simulink model "PV_validation"  (R2020a)
settings: Solver=VariableStepAuto  StartTime=0.0  StopTime=10  RelTol=1e-3
values from neighbouring files (symbols this model uses):
  Ts = 10e-6    (= 1e-05)    [run_validation.m]    (also in tune_inverter_GFL.m; tune_inverter_PV_GFL.m; tune_iter_GFL.m = tsim(2)-tsim(1); tune_iter_PV_GFL.m = tsim(2)-tsim(1))
libraries: powerlib x6, libFC_PV x1
settings Model: SimulationMode=accelerator  Creator=pkoralew  LastModifiedBy=pkoralew

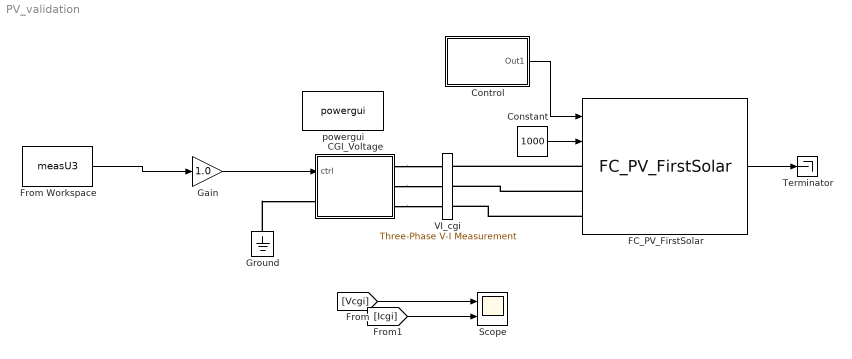
== system PV_validation ==
  CGI_Voltage : Subsystem
  Constant : Constant  Value=1000
  Control : Subsystem
  FC_PV_FirstSolar : libFC_PV/FC_PV_FirstSolar  EnArray=off  Ts=Ts  cc_kp=-1  cc_Ti=-1  pll_kp=-1  pll_ki=-1
  From Workspace : FromWorkspace  VariableName=measU3  SampleTime=Ts
  Gain : Gain  Gain=1.0
  Ground : powerlib/Elements/Ground  LConnTagsString=a
  Scope : Scope  NumInputPorts=2
  Terminator : Terminator
  VI_cgi : powerlib/Measurements/Three-Phase V-I Measurement  VoltageMeasurement=phase-to-ground  SetLabelV=on  LabelV=Vcgi  Vpu=off  VpuLL=off  CurrentMeasurement=yes  SetLabelI=on  LabelI=Icgi  Ipu=off  Pbase=100e6  Vbase=500e3  OutputType=Complex  PhasorSimulation=off  PSBequivalent=0
  powergui : powerlib/powergui  Priority=1  SimulationMode=Discrete  SampleTime=Ts  frequency=60  Iterations=50  frequencyindice=0  Pbase=100e6  ErrMax=1e-4  UnitsV=kV  UnitsW=MW  buscounter=0  FunctionMessages=off  echomessages=off  EnableUseOfTLC=off  CurrentSourceSwitches=off  DisableSnubberDevices=off  DisableRonSwitches=off  DisableVfSwitches=off  DisplayEquations=off  AutomaticDiscreteSolvers=off  SolverType=Tustin/Backward Euler (TBE)  Interpol=off  ExternalGateDelay=off  methode=off  Ts=100  x0status=blocks  SPID=on  SwTol=0  HookPort=off  NonlinearTolerance=1e-4  nMaxIteration=100  ContinueOnMaxIteration=off  RestoreLinks=warning  ResistiveCurrentMeasurement=off  Frange=[0:2:500]  Ylog=off  Xlog=on  ShowGrid=off  save=off  variable=ZData  structure=0  ZoomFFT=off  StartTime=0.0  cycles=1  DisplayStyle=1  fundamental=60  FreqAxis=off  MaxFrequency=1000  frequencyindicesteady=1  RmsSteady=1  display=off
  wires:
  From Workspace/1 -> Gain/1
  [Icgi] -> Scope/2
  FC_PV_FirstSolar/1 -> Terminator/1
  Control/1(Out1) -> FC_PV_FirstSolar/1
  [Vcgi] -> Scope/1
  Gain/1 -> CGI_Voltage/1(ctrl)
  Constant/1 -> FC_PV_FirstSolar/2
  connections:
  Ground/LConn1 -- CGI_Voltage/LConn1
  CGI_Voltage/RConn1 -- VI_cgi/LConn1
  CGI_Voltage/RConn2 -- VI_cgi/LConn2
  CGI_Voltage/RConn3 -- VI_cgi/LConn3
  FC_PV_FirstSolar/LConn2 -- VI_cgi/RConn2
  FC_PV_FirstSolar/LConn1 -- VI_cgi/RConn1
  FC_PV_FirstSolar/LConn3 -- VI_cgi/RConn3

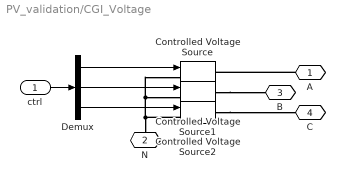
== system PV_validation/CGI_Voltage ==
  ctrl : Inport
  Controlled Voltage Source : powerlib/Electrical Sources/Controlled Voltage Source  Initialize=on  Source_Type=AC  Amplitude=0  Phase=0  Frequency=0  Measurements=None
  Controlled Voltage Source1 : powerlib/Electrical Sources/Controlled Voltage Source  Initialize=on  Source_Type=AC  Amplitude=0  Phase=0  Frequency=0  Measurements=None
  Controlled Voltage Source2 : powerlib/Electrical Sources/Controlled Voltage Source  Initialize=on  Source_Type=AC  Amplitude=0  Phase=0  Frequency=0  Measurements=None
  Demux : Demux  Outputs=3
  A : PMIOPort  Side=Right
  N : PMIOPort  Port=2  Side=Left
  B : PMIOPort  Port=3  Side=Right
  C : PMIOPort  Port=4  Side=Right
  wires:
  Demux/1 -> Controlled Voltage Source/1
  Demux/2 -> Controlled Voltage Source1/1
  Demux/3 -> Controlled Voltage Source2/1
  ctrl/1 -> Demux/1
  connections:
  A/RConn1 -- Controlled Voltage Source/RConn1
  Controlled Voltage Source2/LConn1 -- Controlled Voltage Source/LConn1 -- Controlled Voltage Source1/LConn1 -- N/RConn1
  Controlled Voltage Source1/RConn1 -- B/RConn1
  Controlled Voltage Source2/RConn1 -- C/RConn1

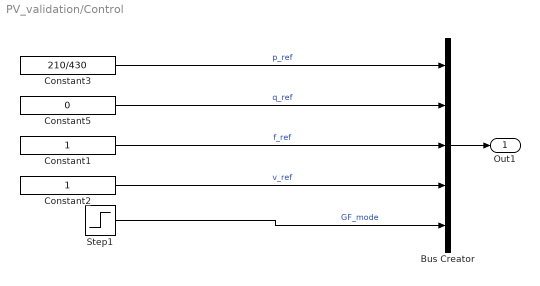
== system PV_validation/Control ==
  Bus Creator : BusCreator  Inputs=5
  Constant1 : Constant  SampleTime=-1
  Constant2 : Constant  SampleTime=-1
  Constant3 : Constant  Value=210/430  SampleTime=-1
  Constant5 : Constant  Value=0  SampleTime=-1
  Step1 : Step  Time=1000
  Out1 : Outport
  wires:
  Constant2/1 -> Bus Creator/4  "v_ref"
  Bus Creator/1 -> Out1/1
  Constant1/1 -> Bus Creator/3  "f_ref"
  Step1/1 -> Bus Creator/5  "GF_mode"
  Constant5/1 -> Bus Creator/2  "q_ref"
  Constant3/1 -> Bus Creator/1  "p_ref"
